simulink model "MRAC"  (R2021b)
settings: Solver=VariableStepAuto  StartTime=0.0  StopTime=30  RelTol=1e-3
settings Model: Creator=cesar  LastModifiedBy=cesar

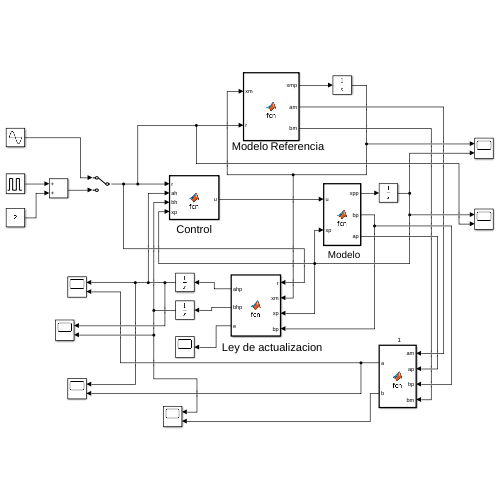
[thumbnail: Simulink's stored preview of the top-level diagram]
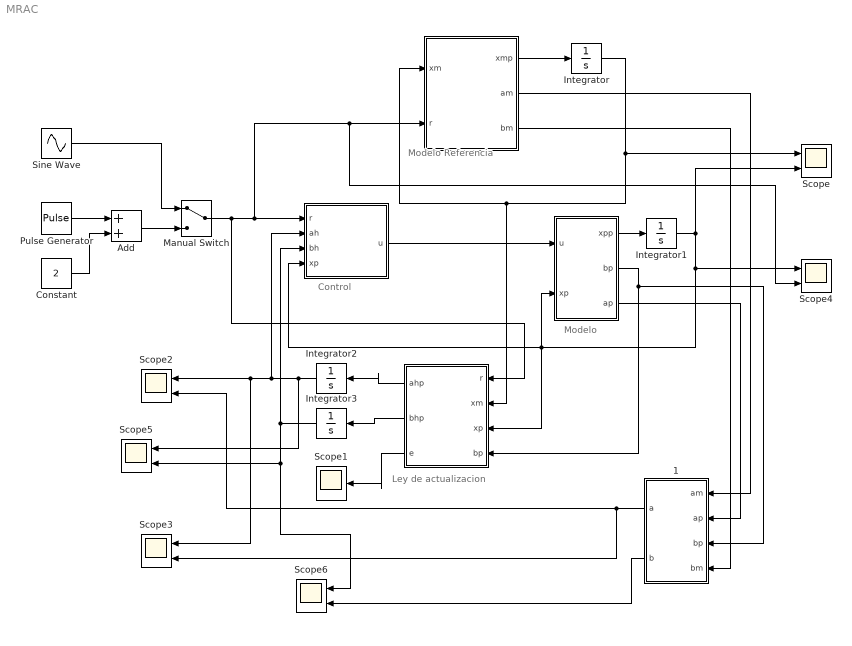
== system MRAC ==
  note: Modelo
  note: Modelo Referencia
  note: Control
  note: Ley de actualizacion
  "  " : MATLAB Function  TreatAsAtomicUnit=on
  "   " : MATLAB Function  TreatAsAtomicUnit=on
  "    " : MATLAB Function  TreatAsAtomicUnit=on
  "     " : MATLAB Function  TreatAsAtomicUnit=on
  "  1" : MATLAB Function  TreatAsAtomicUnit=on
  Add : Sum
  Constant : Constant  Value=2
  Integrator{,1..3} (4 alike) : Integrator
  Manual Switch : ManualSwitch
  Pulse Generator : DiscretePulseGenerator  PulseType=Time based  Period=10  PulseWidth=5
  Scope{,2..6} (6 alike) : Scope  NumInputPorts=2
  Scope1 : Scope
  Sine Wave : Sin  Amplitude=2  Frequency=4  SampleTime=0
  wires:
  "  "/1(xpp) -> Integrator1/1
  "   "/1(xmp) -> Integrator/1
  Integrator/1 -> "   "/1(xm), "    "/2(xm), Scope/1
  Integrator1/1 -> "    "/3(xp), "     "/4(xp), "  "/2(xp), Scope4/1, Scope/2
  "     "/1(u) -> "  "/1(u)
  Pulse Generator/1 -> Add/1
  Constant/1 -> Add/2
  Manual Switch/1 -> "    "/1(r), Scope4/2, "   "/2(r), "     "/1(r)
  Add/1 -> Manual Switch/2
  "    "/1(ahp) -> Integrator2/1
  "    "/2(bhp) -> Integrator3/1
  Integrator2/1 -> Scope5/1, Scope3/1, Scope2/1, "     "/2(ah)
  Integrator3/1 -> "     "/3(bh), Scope6/1, Scope5/2
  "  "/2(bp) -> "  1"/3(bp), "    "/4(bp)
  "    "/3(e) -> Scope1/1
  "  "/3(ap) -> "  1"/2(ap)
  "   "/2(am) -> "  1"/1(am)
  "   "/3(bm) -> "  1"/4(bm)
  "  1"/1(a) -> Scope3/2, Scope2/2
  Sine Wave/1 -> Manual Switch/1
  "  1"/2(b) -> Scope6/2

== matlab function MRAC/    ==
  data: xm input; xmp output; r input; am output; bm output
function [xmp, am,bm]  = fcn(xm,r)
am = -4;
bm = 5;

xmp = am*xm + bm*r;

== matlab function MRAC/   ==
  data: u input; xp input; xpp output; bp output; ap output
function [xpp,bp,ap]  = fcn(u,xp)
ap = 8;
%ap = sin(8);
bp = 5;

xpp = ap*xp + bp*u;

== matlab function MRAC/      ==
  data: r input; ah input; bh input; xp input; u output
function u  = fcn(r,ah,bh,xp)

u = ah*xp + bh*r;

== matlab function MRAC/     ==
  data: r input; xm input; xp input; ahp output; bhp output; bp input; e output
function [ahp, bhp,e]  = fcn(r,xm,xp,bp)
%Error de seguimiento
e = xp - xm;

ahp = -sign(bp)*e*xp;
bhp = -sign(bp)*e*r;

== matlab function MRAC/  1 ==
  data: am input; ap input; a output; b output; bp input; bm input
function [a,b]  = fcn(am,ap,bp,bm)



a = (am - ap)/bp;
b = bm/bp;
